simulink model "test_disturb"  (R2024b)
settings: Solver=VariableStepAuto  StartTime=0.0  StopTime=10.0  RelTol=1e-3
undefined symbols (not defined in the file): gain
libraries: cstblocks x2
settings Model: Creator=1163390615  LastModifiedBy=1163390615

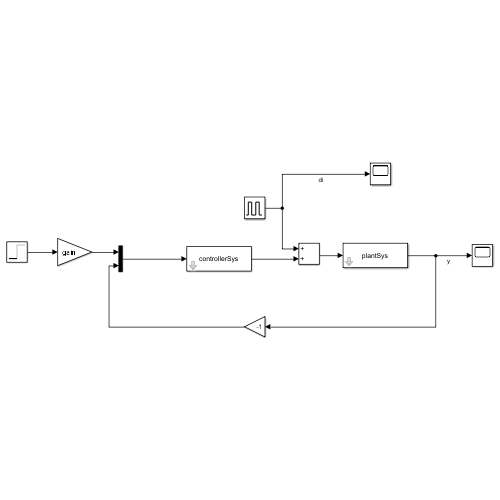
[thumbnail: Simulink's stored preview of the top-level diagram]
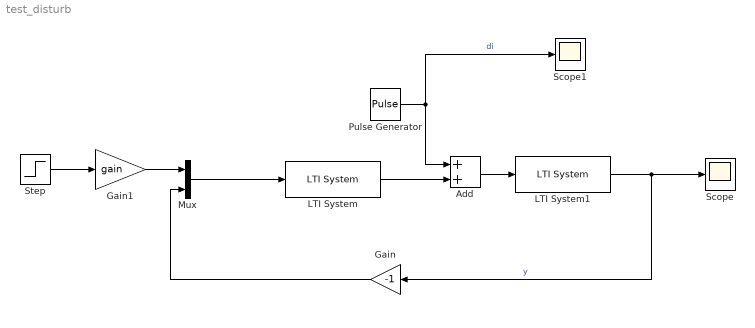
== system test_disturb ==
  Add : Sum
  Gain : Gain  Gain=-1
  Gain1 : Gain  Gain=gain
  LTI System : cstblocks/LTI System  sys=controllerSys  IC=[]  PadeOrder=0
  LTI System1 : cstblocks/LTI System  sys=plantSys  IC=[]  PadeOrder=0
  Mux : Mux  Inputs=2
  Pulse Generator : DiscretePulseGenerator  PulseType=Time based  Period=3  PulseWidth=5
  Scope : Scope
  Scope1 : Scope
  Step : Step  SampleTime=0
  wires:
  Step/1 -> Gain1/1
  Gain/1 -> Mux/2
  LTI System/1 -> Add/2
  LTI System1/1 -> Gain/1, Scope/1  "y"
  Mux/1 -> LTI System/1
  Gain1/1 -> Mux/1
  Pulse Generator/1 -> Add/1, Scope1/1  "di"
  Add/1 -> LTI System1/1
